simulink model "Nugraha_Setya_Ardi_10714522_952033"  (R2020b)
settings: Solver=ode15s  StartTime=0.0  StopTime=1000
undefined symbols (not defined in the file): deg, s
libraries: sharedtransform x1
settings Model: SimulationMode=rapid-accelerator  Creator=nugra  LastModifiedBy=nugra
settings SolverCC: ZeroCrossAlgorithm=Adaptive

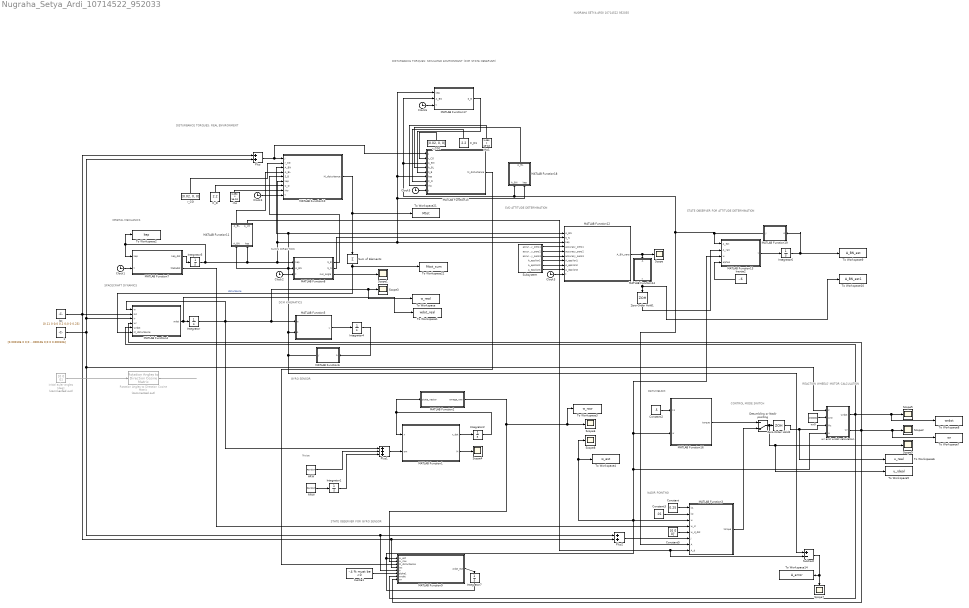
== system Nugraha_Setya_Ardi_10714522_952033 ==
  note: Noise
  note: GYRO SENSOR
  note: NADIR POINTNG
  note: DETUMBLING
  note: REACTION WHEELS'
      | MOTOR CALCULATION
  note: DCM KINEMATICS
  note: DISTURBANCE TORQUES:
      | REAL ENVIRONMENT
  note: ORBITAL MECHANICS
  note: SUN'S DIRECTION
  note: SPACECRAFT DYNAMICS
  note: CONTROL MODE
      | SWITCH
  note: STATE OBSERVER FOR
      | GYRO SENSOR
  note: STATE OBSERVER FOR
      | ATTITUDE DETERMINATION
  note: DISTURBANCE TORQUES:
      | SIMULATED ENVIRONMENT
      | (FOR STATE OBSERVER)
  note: NUGRAHA SETYA ARDI
      | 10714522
      | 952035
  note: SVD ATTITUDE DETERMINATION
  ARW : RandomNumber  Variance=(1/4*deg2rad([0.2 0.2 0.2]/sqrt(3600))).^2 %[0.2 deg/s^.5]  SampleTime=1/1000
  C_D : Constant  Value=2.2
  C_D1 : Constant  Value=2.2
  Clock{1..6} (6 alike) : Clock
  Constant : Constant  Value=0.25
  Constant2 : Constant  Value=.5
  Constant3 : Constant  Value=.01
  Constant5 : Constant  Value=[0 0 0]'
  Detumbling or Nadir pointing : ManualSwitch  CurrentSetting=0
  Inertia1 : Constant  Value=-.4 % must be <0
  Inertia2 : Constant  Value=-.6
  Integrator : Integrator  InitialCondition=deg2rad([5 10 -7])
  Integrator1 : Integrator  InitialCondition=[1/3600 1/3600 1/3600] % [deg/s], i.e. 1 deg/hour
  Integrator2 : Integrator  InitialCondition=[0 0 0 0 0 0]'
  Integrator4 : Integrator  InitialCondition=eye(3,3)
  Integrator5 : Integrator  InitialCondition=[7500, 0.1, deg2rad(10), deg2rad(40), deg2rad(60), 0]
  Integrator6 : Integrator  InitialCondition=zeros(3,3)
  Integrator7 : Integrator  InitialCondition=[0 0 0]
  Ir : Constant  Value=[0.000106 0 0;0 0.000106 0;0 0 0.000106]  VectorParams1D=off
  Isc : Constant  Value=[0.11 0 0;0 0.2 0;0 0 0.23]  VectorParams1D=off
  MATLAB Function1 : MATLAB Function  TreatAsAtomicUnit=on
  MATLAB Function10 : MATLAB Function  TreatAsAtomicUnit=on
  MATLAB Function11 : MATLAB Function  TreatAsAtomicUnit=on
  MATLAB Function12 : MATLAB Function  TreatAsAtomicUnit=on
  MATLAB Function13 : MATLAB Function  TreatAsAtomicUnit=on
  MATLAB Function14 : MATLAB Function  TreatAsAtomicUnit=on
  MATLAB Function15 : MATLAB Function  TreatAsAtomicUnit=on
  MATLAB Function16 : MATLAB Function  TreatAsAtomicUnit=on
  MATLAB Function17 : MATLAB Function  TreatAsAtomicUnit=on
  MATLAB Function18 : MATLAB Function  TreatAsAtomicUnit=on
  MATLAB Function19 : MATLAB Function  TreatAsAtomicUnit=on
  MATLAB Function2 : MATLAB Function  TreatAsAtomicUnit=on
  MATLAB Function3 : MATLAB Function  TreatAsAtomicUnit=on
  MATLAB Function4 : MATLAB Function  TreatAsAtomicUnit=on
  MATLAB Function5 : MATLAB Function  TreatAsAtomicUnit=on
  MATLAB Function6 : MATLAB Function  TreatAsAtomicUnit=on
  MATLAB Function7 : MATLAB Function  TreatAsAtomicUnit=on
  MATLAB Function8 : MATLAB Function  TreatAsAtomicUnit=on
  MATLAB Function9 : MATLAB Function  TreatAsAtomicUnit=on
  Plus : Sum
  Plus1 : Sum  Inputs=+++
  Plus2 : Sum
  RRW : RandomNumber  Variance=(1/4*deg2rad([0.3 0.3 0.3]/3600)).^2 % [0.3 deg/s^1.5]  SampleTime=1/1000
  Rotation Angles to Direction Cosine Matrix : sharedtransform/Rotation Angles to Direction Cosine Matrix  Commented=on  rotationOrder=XYZ  aMode=aMode
      settings: SourceProductBaseCode=AE,PW,MT,UV,VE,VP
  Scope{,1..9} (10 alike) : Scope
  Subsystem : Subsystem
  Subtract : Sum  Inputs=+-
  Sum of Elements : Sum  Inputs=+  CollapseMode=Specified dimension  CollapseDim=2
  To Workspace : ToWorkspace  VariableName=w_real  SaveFormat=Structure With Time  SampleTime=-1
  To Workspace1 : ToWorkspace  VariableName=wdot_real  SaveFormat=Structure With Time  SampleTime=-1
  To Workspace10 : ToWorkspace  VariableName=A_BN_est1  SaveFormat=Timeseries  SampleTime=-1
  To Workspace14 : ToWorkspace  VariableName=A_error  SaveFormat=Structure With Time  SampleTime=-1
  To Workspace2 : ToWorkspace  VariableName=kep  SaveFormat=Timeseries  SampleTime=-1
  To Workspace21 : ToWorkspace  VariableName=Mtot  SaveFormat=Structure With Time  SampleTime=-1
  To Workspace22 : ToWorkspace  VariableName=Mtot_sum  SaveFormat=Structure With Time  SampleTime=-1
  To Workspace3 : ToWorkspace  VariableName=w_raw  SaveFormat=Structure With Time  SampleTime=-1
  To Workspace4 : ToWorkspace  VariableName=w_est  SaveFormat=Structure With Time  SampleTime=-1
  To Workspace5 : ToWorkspace  VariableName=u_ideal  SaveFormat=Structure With Time  SampleTime=-1
  To Workspace6 : ToWorkspace  VariableName=u_real  SaveFormat=Structure With Time  SampleTime=-1
  To Workspace7 : ToWorkspace  VariableName=wr  SaveFormat=Structure With Time  SampleTime=-1
  To Workspace8 : ToWorkspace  VariableName=wrdot  SaveFormat=Structure With Time  SampleTime=-1
  To Workspace9 : ToWorkspace  VariableName=A_BN_est  SaveFormat=Timeseries  SampleTime=-1
  Zero-Order Hold1 : ZeroOrderHold  SampleTime=0.01
  Zero-Order Hold2 : ZeroOrderHold  SampleTime=0.01
  initial euler angles [deg] : Constant  Commented=on  Value=[0 0 0]
  r_CG : Constant  Value=[0.02, 0, 0]'
  r_CG1 : Constant  Value=[0.02, 0, 0]'
  rho : Constant  Value=1.454 * 1e-13
  rho1 : Constant  Value=1.454 * 1e-13
  wr and wrdot calculation : Subsystem
  wr0 : Constant  Value=[0;0;0]
  wires:
  MATLAB Function4/1(wdot) -> To Workspace1/1, Integrator/1
  Isc/1 -> Plus/1, MATLAB Function9/4(Isc), Plus2/2, MATLAB Function4/2(Isc)
  Ir/1 -> Plus2/1, MATLAB Function9/5(Ir), wr and wrdot calculation/1(Ir), Plus/2, MATLAB Function4/3(Ir)
  MATLAB Function5/1(y) -> Integrator4/1
  Integrator4/1 -> MATLAB Function6/1(A)
  Clock1/1 -> MATLAB Function7/2(t)
  MATLAB Function7/1(kep_dot) -> Integrator5/1
  Clock2/1 -> MATLAB Function8/3(t)
  Subsystem/2(accuracy_sens2) -> MATLAB Function12/5(accuracy_sens2)
  MATLAB Function6/1(y) -> Subtract/1, MATLAB Function11/1(A_BN), MATLAB Function10/3(A_BN), MATLAB Function12/1(A_BN), MATLAB Function8/2(A_BN), MATLAB Function5/2(A)
  Subsystem/1(accuracy_sens1) -> MATLAB Function12/4(accuracy_sens1)
  MATLAB Function8/2(S_N) -> MATLAB Function12/2(S_N)
  Integrator5/1 -> MATLAB Function11/2(kep), MATLAB Function8/1(kep), MATLAB Function10/6(kep), MATLAB Function12/3(kep), MATLAB Function18/2(kep), MATLAB Function17/1(kep), MATLAB Function15/6(kep), MATLAB Function7/1(kep), To Workspace2/1
  Clock3/1 -> MATLAB Function12/10(t)
  MATLAB Function8/1(S_B) -> MATLAB Function10/5(S_B)
  Clock4/1 -> MATLAB Function10/9(t)
  C_D/1 -> MATLAB Function10/7(C_D)
  rho/1 -> MATLAB Function10/8(rho)
  r_CG/1 -> MATLAB Function10/2(r_CG)
  Plus/1 -> MATLAB Function15/1(J), MATLAB Function10/1(J)
  MATLAB Function11/1(A_BL) -> MATLAB Function10/4(A_BL)
  Integrator1/1 -> Plus1/3
  MATLAB Function1/2(M) -> Scope4/1
  MATLAB Function1/1(x_dot) -> Integrator2/1
  RRW/1 -> Integrator1/1
  Integrator/1 -> MATLAB Function5/1(w), To Workspace/1, Scope3/1, Plus1/1, MATLAB Function4/1(w)
  ARW/1 -> Plus1/2
  Plus1/1 -> MATLAB Function1/2(om)
  Constant2/1 -> MATLAB Function16/1(k1)
  MATLAB Function16/1(torque) -> Detumbling or Nadir pointing/1
  wr0/1 -> wr and wrdot calculation/2(wr0)
  wr and wrdot calculation/1(wrdot) -> MATLAB Function9/7(wrdot), To Workspace8/1, Scope5/1, MATLAB Function4/5(wrdot)
  wr and wrdot calculation/2(wr) -> MATLAB Function9/8(wr), To Workspace7/1, Scope2/1, MATLAB Function4/4(wr)
  Integrator2/1 -> MATLAB Function1/1(x), MATLAB Function2/1(state_vector)
  MATLAB Function8/3(sun_angle) -> Scope1/1
  Constant/1 -> MATLAB Function3/1(k1)
  Constant3/1 -> MATLAB Function3/2(k2)
  MATLAB Function11/2(A_LN) -> Subtract/2, MATLAB Function3/8(A_d)
  MATLAB Function7/2(thetadot) -> MATLAB Function3/4(w_d)
  Constant5/1 -> MATLAB Function3/5(w_d_dot)
  MATLAB Function3/1(torque) -> Detumbling or Nadir pointing/2
  Plus2/1 -> MATLAB Function3/6(J)
  Detumbling or Nadir pointing/1 -> To Workspace5/1, Scope9/1, Zero-Order Hold2/1
  Subtract/1 -> Scope7/1, To Workspace14/1
  MATLAB Function2/1(omega_raw) -> MATLAB Function9/2(w_raw), To Workspace3/1, Scope6/1
  Zero-Order Hold1/1 -> MATLAB Function13/2(A_raw)
  Zero-Order Hold2/1 -> To Workspace6/1, wr and wrdot calculation/3(Mc)
  MATLAB Function9/1(wdot_est) -> Integrator7/1
  Inertia1/1 -> MATLAB Function9/6(alpha1)
  MATLAB Function10/1(M_disturbance) -> To Workspace21/1, Sum of Elements/1
  MATLAB Function13/1(y) -> Integrator6/1
  Inertia2/1 -> MATLAB Function13/4(alpha1)
  Clock5/1 -> MATLAB Function15/9(t)
  r_CG1/1 -> MATLAB Function15/2(r_CG)
  C_D1/1 -> MATLAB Function15/7(C_D)
  rho1/1 -> MATLAB Function15/8(rho)
  Clock6/1 -> MATLAB Function17/3(t)
  MATLAB Function17/1(S_B) -> MATLAB Function15/5(S_B)
  MATLAB Function18/1(A_BL) -> MATLAB Function15/4(A_BL)
  MATLAB Function15/1(M_disturbance) -> MATLAB Function9/3(M_disturbance)
  Subsystem/3(accuracy_sens3) -> MATLAB Function12/6(accuracy_sens3)
  Subsystem/4(A_epsilon1) -> MATLAB Function12/7(A_epsilon1)
  Subsystem/5(A_epsilon2) -> MATLAB Function12/8(A_epsilon2)
  Subsystem/6(A_epsilon3) -> MATLAB Function12/9(A_epsilon3)
  Integrator7/1 -> wr and wrdot calculation/4(w), MATLAB Function13/3(w), MATLAB Function16/2(w), MATLAB Function3/3(w), To Workspace4/1, Scope8/1, MATLAB Function9/1(w_est)
  MATLAB Function12/1(A_BN_sens) -> Scope/1, MATLAB Function14/1(A)
  Integrator6/1 -> To Workspace9/1, MATLAB Function19/1(A)
  MATLAB Function14/1(y) -> Zero-Order Hold1/1, To Workspace10/1
  Sum of Elements/1 -> MATLAB Function4/6(M_disturbance), To Workspace22/1  "disturbance"
  Rotation Angles to Direction Cosine Matrix/1 -> ?
  initial euler angles [deg]/1 -> Rotation Angles to Direction Cosine Matrix/1
  MATLAB Function19/1(y) -> MATLAB Function3/7(A), MATLAB Function18/1(A_BN), MATLAB Function17/2(A_BN), MATLAB Function15/3(A_BN), MATLAB Function13/1(A_est)

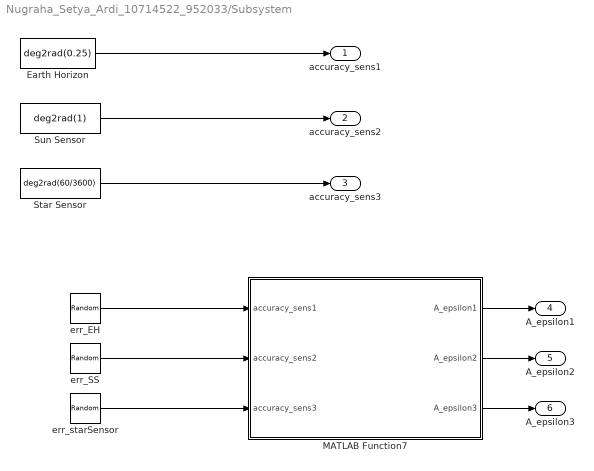
== system Nugraha_Setya_Ardi_10714522_952033/Subsystem ==
  Earth Horizon : Constant  Value=deg2rad(0.25)
  MATLAB Function7 : MATLAB Function  TreatAsAtomicUnit=on
  Star Sensor : Constant  Value=deg2rad(60/3600)
  Sun Sensor : Constant  Value=deg2rad(1)
  err_EH : RandomNumber  Variance=(1/4*deg2rad([0.25 0.25 0.25])).^2  Seed=[1 2 3]  SampleTime=1/100
  err_SS : RandomNumber  Variance=(1/4*deg2rad([1 1 1])).^2  Seed=[4 5 6]  SampleTime=1/100
  err_starSensor : RandomNumber  Variance=(1/4*deg2rad([60/3600 60/3600 60/3600])).^2  Seed=[4 5 6]  SampleTime=1/4
  accuracy_sens1 : Outport
  accuracy_sens2 : Outport  Port=2
  accuracy_sens3 : Outport  Port=3
  A_epsilon1 : Outport  Port=4
  A_epsilon2 : Outport  Port=5
  A_epsilon3 : Outport  Port=6
  wires:
  MATLAB Function7/1(A_epsilon1) -> A_epsilon1/1
  MATLAB Function7/2(A_epsilon2) -> A_epsilon2/1
  Earth Horizon/1 -> accuracy_sens1/1
  Sun Sensor/1 -> accuracy_sens2/1
  err_SS/1 -> MATLAB Function7/2(accuracy_sens2)
  err_EH/1 -> MATLAB Function7/1(accuracy_sens1)
  Star Sensor/1 -> accuracy_sens3/1
  err_starSensor/1 -> MATLAB Function7/3(accuracy_sens3)
  MATLAB Function7/3(A_epsilon3) -> A_epsilon3/1

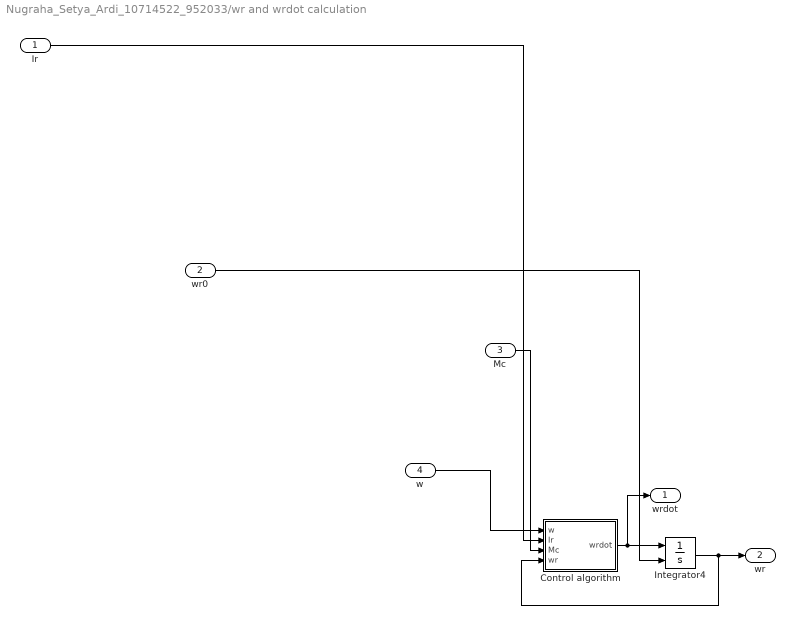
== system Nugraha_Setya_Ardi_10714522_952033/wr and wrdot calculation ==
  Ir : Inport
  wr0 : Inport  Port=2
  Mc : Inport  Port=3
  w : Inport  Port=4
  Control algorithm : MATLAB Function  TreatAsAtomicUnit=on
  Integrator4 : Integrator  InitialConditionSource=external
  wrdot : Outport
  wr : Outport  Port=2
  wires:
  Control algorithm/1(wrdot) -> wrdot/1, Integrator4/1
  Ir/1 -> Control algorithm/2(Ir)
  wr0/1 -> Integrator4/2
  Mc/1 -> Control algorithm/3(Mc)
  w/1 -> Control algorithm/1(w)
  Integrator4/1 -> Control algorithm/4(wr), wr/1

== matlab function Nugraha_Setya_Ardi_10714522_952033/MATLAB Function8 ==
  data: S_B output; S_N output; kep input; sun_angle output; A_BN input; t input
function [ S_B, S_N, sun_angle] = sun_direction(kep, A_BN, t)
% kep = [a e i om, Om, th]
a  = kep(1);
e  = kep(2);
i  = kep(3);
om = kep(4);
Om = kep(5);
th = kep(6);

R = a*(1-e^2) / (1+e*cos(th));
r_N = R * [cos(th);
           sin(th)*cos(i);
           sin(th)*sin(i)];
r_B = A_BN * r_N;

R_s = 149597870.691; % 1AU [km]
mu_s = 132712440017.987;
n_s  = sqrt(mu_s/R_s^3);

epsilon = deg2rad(23.45);
% Sun direction w.r.t. S/C ~ Sun direction w.r.t. Earth
S_N = R_s * [cos(n_s*t), sin(n_s*t)*cos(epsilon), sin(n_s*t)*sin(epsilon)]';
S_B = A_BN*S_N;

sun_angle = acos(complex(dot(r_B, S_B)/(norm(r_B)*norm(S_B))));

== matlab function Nugraha_Setya_Ardi_10714522_952033/MATLAB Function9 ==
  data: w_est input; w_raw input; M_disturbance input; wdot_est output; Isc input; Ir input; alpha1 input; wrdot input; wr input
function wdot_est = stateObserbver(w_est,w_raw,M_disturbance,Isc,Ir,alpha1,wrdot,wr)
% 
% 
% % Moments of Inertia [kg*m^2]
% % (12U Cubesat)
% J1 = J(1,1);
% J2 = J(2,2);
% J3 = J(3,3);
% 
% C1 = (J2-J3)/J1;
% C2 = (J3-J1)/J2;
% C3 = (J1-J2)/J3;
% 
% 
% w_est_dot = zeros(3,1);
% w_est_dot(1) = C1 * w_est(2)*w_est(3) + u_tot(1)/J1 + alpha1*(w_est(1) - w_raw(1));
% w_est_dot(2) = C2 * w_est(1)*w_est(3) + u_tot(2)/J2 + alpha1*(w_est(2) - w_raw(2));
% w_est_dot(3) = C3 * w_est(1)*w_est(2) + u_tot(3)/J3 + alpha1*(w_est(3) - w_raw(3));

wdot_est = inv(Isc)*(M_disturbance - cross(w_est,(Isc*w_est)) - Ir*wrdot - cross(w_est,(Ir*wr))) + alpha1*(w_est-w_raw);

== matlab function Nugraha_Setya_Ardi_10714522_952033/MATLAB Function10 ==
  data: J input; r_CG input; A_BN input; M_disturbance output; A_BL input; S_B input; kep input; C_D input; rho input; t input
function M_disturbance    = disturbanceTorques(J, r_CG, A_BN, A_BL, S_B, kep, C_D, rho, t)

G = 6.67408e-11;
m_E = 5.972e+24;
a  = kep(1);    e  = kep(2);    i = kep(3);
OM = kep(4);    om = kep(5);    th = kep(6);
R_equat = 6371e+3; % [m]
p = a*(1-e^2);
R = p / (1+e*cos(th)) * 1e+3; % [m]

% Moments of Inertia [kg*m^2]
% (12U Cubesat)
J1 = J(1,1);
J2 = J(2,2);
J3 = J(3,3);

C1 = (J2-J3)/J1;
C2 = (J3-J1)/J2;
C3 = (J1-J2)/J3;
%% Gravity Gradient Torque
c = A_BL * [1;0;0];

M_GG = [- 3*G*m_E/R^3 *C1* c(3)*c(2);
        - 3*G*m_E/R^3 *C2* c(1)*c(3);
        - 3*G*m_E/R^3 *C3* c(2)*c(1)];
                      
%% SRP Torque @ 600 Km (Direct Solar Rad. + Sun Rad. Reflected by Earth + Earth Rad.)
F_e = 1358 + 580 + 143.4; % [W/m^2]
P = F_e / (3*1e+8);

N_body = 6; % # main body surfaces
N_SP = 4; % # solar panel surfaces

U = 0.1; % 1U length

N = zeros(N_body+N_SP,3);
A = zeros(N_body+N_SP,1);
r = zeros(N_body+N_SP,3);
n1 = [1 0 0];  n2 = [0 1 0];  n3 = [0 0 1];
% S/C Main Body: Normals, Surface Coefficients, Areas
N(1,:) = n1;    N(2,:) = n2;     N(3,:) = n3;
N(4,:) = -n1;   N(5,:) = -n2;   N(6,:) = -n3;
rho_s_body = .5;     rho_d_body = .1;
A(1:N_body) = [4 8 8 4 8 8]*U^2; % [m^2]

% Solar Panels: Normals, Surface Coefficients, Areas
N(7,:) = n1;    N(8,:) = -n1;   N(9,:) = n1;    N(10,:) = -n1;
rho_s_SP = .5;     rho_d_SP = .1;
A(N_body+1:N_body+N_SP) = [8 8 8 8]*U^2; % [m^2]

% L.u.c. a RF centered @ Geometric Center of S/C::
% we will use it to define the coordinates of each surface's center
% along w/ the coordinates of th CG w.r.t. GC
r(1,:) = [2 0 0]*U;  r(2,:) = [0 1 0]*U;  r(3,:) = [0 0 1]*U;
r(4,:) = [-2 0 0]*U; r(5,:) = [0 -1 0]*U; r(6,:) = [0 0 -1]*U;
r(7,:) = [-2 3 0]*U;   r(8,:)  = [-2 -3 0]*U;
r(9,:) = [-2 3 0]*U;   r(10,:) = [-2 -3 0]*U;

S_B_norm = S_B / norm(S_B);

M_SRP = zeros(3,1);
for k = 1:N_body+N_SP
    if k <= N_body
        rho_s = rho_s_body;     rho_d = rho_d_body;
    else
        rho_s = rho_s_SP;       rho_d = rho_d_SP;
    end
    
    n_k = N(k,:)';
    F_k = - P*A(k)*dot(S_B_norm,n_k) * ( (1-rho_s)*S_B_norm + (2*rho_s*dot(S_B_norm,n_k)+2/3*rho_d)*n_k );
    
    if dot(S_B_norm, n_k) > 0
        r_k = (r(k,:) - r_CG')';
        M_SRP_k = cross(r_k, F_k);
    else
        M_SRP_k = zeros(3,1);
    end
    
    M_SRP = M_SRP + M_SRP_k;
        
end

%% Air-Drag Torque

w_E = 2*pi/(23*3600 + 56*60 + 4.09); % Earth's angular rate [rad/s]
mu_E = 398600.433; % [km^3/s^2]



% Rotation matrices: Earth-Centered Inertial --> Perifocal   (ECI->PF)
R_om = [cos(om)  sin(om)    0   ;
        -sin(om) cos(om)    0   ;
           0        0       1   ];
       
R_i  = [   1        0       0   ;
           0     cos(i)   sin(i);
           0    -sin(i)   cos(i)];
       
R_OM = [cos(OM)  sin(OM)    0   ;
        -sin(OM) cos(OM)    0   ;
           0        0       1   ];
    
R313 = R_om * R_i * R_OM; % ECI --> PF


R_PF = R * [cos(th), sin(th), 0]';
v_PF = sqrt(mu_E/p) * [-sin(th), (e+cos(th)), 0]';
% PF --> ECI
r_ECI = R313'* R_PF;
v_ECI = R313'* v_PF;


v_rel_N = v_ECI + cross([0 0 w_E]', r_ECI);

v_rel_B = A_BN*v_rel_N; % Relative atmosphere velocity (@body frame)
v_rel_B_unit = v_rel_B / norm(v_rel_B);


M_drag = zeros(3,1);
for k = 1:N_body+N_SP
    
    n_k = N(k,:)';
    F_k = - .5 * C_D * rho * norm(v_rel_B)^2 * dot(n_k,v_rel_B_unit) * A(k) * v_rel_B_unit;
    
    
    if dot(S_B_norm, n_k) > 0
        r_k = (r(k,:) - r_CG')';
        M_drag_k = cross(r_k, F_k);
    else
        M_drag_k = zeros(3,1);
    end
    
    M_drag = M_drag + M_drag_k;
        
end

%% Magnetic Torque
g10 = -29615e-9;  g11 = -1728e-9;   h11 = 5186e-9;
H0 = sqrt(g10^2 + g11^2 + h11^2);
m = [sind(11.5)*cos(w_E*t);
     sind(11.5)*sin(w_E*t);
     cosd(11.5)];
r_N = R * [cos(th);
           sin(th)*cos(i);
           sin(th)*sin(i)];
       
% Magnetic field vector
b_N = R_equat^3*H0/R^3 * (3*dot(m/norm(m),r_N/norm(r_N))*r_N/norm(r_N) - m/norm(m));
b_B = A_BN * b_N;

% Parasitic magnetic torque
M_magn = cross(m, b_B);

M_disturbance = [M_SRP(:), M_magn(:), M_GG(:)];

== matlab function Nugraha_Setya_Ardi_10714522_952033/MATLAB Function11 ==
  data: A_BN input; A_BL output; kep input; A_LN output
function [A_BL, A_LN] = fcn(A_BN, kep)

i  = kep(3);
Om = kep(4)
w = kep(5);
th = kep(6);


A_1 = [ cos(th+w) sin(th+w) 0;
        -sin(th+w) cos(th+w) 0;
          0         0    1];
A_2 = [1      0     0;
       0   cos(i) sin(i);
       0  -sin(i) cos(i)];
A_3 = [cos(Om) sin(Om) 0;-sin(Om) cos(Om) 0;0 0 1];
A_LN = A_1*A_2*A_3;

A_BL = A_BN*A_LN';

== matlab function Nugraha_Setya_Ardi_10714522_952033/MATLAB Function12 ==
  data: A_BN input; A_BN_sens output; S_N input; kep input; accuracy_sens1 input; accuracy_sens2 input; accuracy_sens3 input; A_epsilon1 input; A_epsilon2 input; A_epsilon3 input; t input
function A_BN_sens = sensorModel(A_BN, S_N, kep, accuracy_sens1, accuracy_sens2,accuracy_sens3, A_epsilon1, A_epsilon2,A_epsilon3, t)

i = kep(3);
th = kep(6);

r_N =      [cos(th);
           sin(th)*cos(i);
           sin(th)*sin(i)]; % unit vector that identifies S/C's position w.r.t.
                            % inertial frame centered at Earth
                            
S_N = S_N / norm(S_N);  % unit vector that identifies Sun direction in the
                        % inertial frame
v_N1 = r_N;     
v_N2 = S_N;
v_N3 = [1;0;0]          % fixed star for star sensor
v_B1 = A_epsilon1 * A_BN * v_N1;
v_B2 = A_epsilon2 * A_BN * v_N2;
v_B3 = A_epsilon3 * A_BN * v_N3;

%% SVD algorithm for attitude estimation
prec_sens1 = 1/norm(accuracy_sens1);
prec_sens2 = 1/norm(accuracy_sens2);
prec_sens3 = 1/norm(accuracy_sens3);
alpha = [prec_sens1 prec_sens2 prec_sens3] / (prec_sens1+prec_sens2+prec_sens3); % s.t. sum(alpha) = 1
B = alpha(1)*v_B1*v_N1' + alpha(2)*v_B2*v_N2' + alpha(3)*v_B3*v_N3';
[U,~,V] = svd(B);
M = diag([1, 1, det(U)*det(V)]);
A_BN_sens = U*M*V';

== matlab function Nugraha_Setya_Ardi_10714522_952033/Subsystem/MATLAB Function7 ==
  data: accuracy_sens1 input; A_epsilon1 output; accuracy_sens2 input; A_epsilon2 output; accuracy_sens3 input; A_epsilon3 output
function [A_epsilon1, A_epsilon2, A_epsilon3] = sensor_error(accuracy_sens1, accuracy_sens2, accuracy_sens3)


psi_acc = accuracy_sens1(1);
th_acc  = accuracy_sens1(2);
phi_acc = accuracy_sens1(3);
A_epsilon1 = [cos(psi_acc)*cos(th_acc)  (cos(psi_acc)*sin(th_acc)*sin(phi_acc)+sin(psi_acc)*cos(phi_acc)) (-cos(psi_acc)*sin(th_acc)*cos(phi_acc)+sin(psi_acc)*sin(phi_acc));
                -sin(psi_acc)*cos(th_acc) (-sin(psi_acc)*sin(th_acc)*sin(phi_acc)+cos(psi_acc)*cos(phi_acc))  (sin(psi_acc)*sin(th_acc)*cos(phi_acc)+cos(psi_acc)*sin(phi_acc));
                 sin(th_acc)               -cos(th_acc)*sin(phi_acc)                                           cos(th_acc)*cos(phi_acc)];
             
             

psi_acc = accuracy_sens2(1);
th_acc  = accuracy_sens2(2);
phi_acc = accuracy_sens2(3);
A_epsilon2 = [cos(psi_acc)*cos(th_acc)  (cos(psi_acc)*sin(th_acc)*sin(phi_acc)+sin(psi_acc)*cos(phi_acc)) (-cos(psi_acc)*sin(th_acc)*cos(phi_acc)+sin(psi_acc)*sin(phi_acc));
                -sin(psi_acc)*cos(th_acc) (-sin(psi_acc)*sin(th_acc)*sin(phi_acc)+cos(psi_acc)*cos(phi_acc))  (sin(psi_acc)*sin(th_acc)*cos(phi_acc)+cos(psi_acc)*sin(phi_acc));
                 sin(th_acc)               -cos(th_acc)*sin(phi_acc)                                           cos(th_acc)*cos(phi_acc)];


             
psi_acc = accuracy_sens3(1);
th_acc  = accuracy_sens3(2);
phi_acc = accuracy_sens3(3);
A_epsilon3 = [cos(psi_acc)*cos(th_acc)  (cos(psi_acc)*sin(th_acc)*sin(phi_acc)+sin(psi_acc)*cos(phi_acc)) (-cos(psi_acc)*sin(th_acc)*cos(phi_acc)+sin(psi_acc)*sin(phi_acc));
                -sin(psi_acc)*cos(th_acc) (-sin(psi_acc)*sin(th_acc)*sin(phi_acc)+cos(psi_acc)*cos(phi_acc))  (sin(psi_acc)*sin(th_acc)*cos(phi_acc)+cos(psi_acc)*sin(phi_acc));
                 sin(th_acc)               -cos(th_acc)*sin(phi_acc)                                           cos(th_acc)*cos(phi_acc)];
end

== matlab function Nugraha_Setya_Ardi_10714522_952033/MATLAB Function13 ==
  data: A_est input; A_raw input; w input; y output; alpha1 input
function y = stateObserbver(A_est, A_raw, w, alpha1)
W = [0,    -w(3),  w(2);
     w(3),   0,   -w(1);
    -w(2),  w(1),   0];

A_est_dot = -W * A_est + alpha1*(A_est-A_raw);

y = A_est_dot;

== matlab function Nugraha_Setya_Ardi_10714522_952033/MATLAB Function14 ==
  data: A input; y output
function y = orthonorm(A)

% Recall: for a matrix to be orthonormal it is necessary that
%         det(A)=1  -->  tr(A'A - I) = 0

tol = 1e-7;
k = 0;
while trace(A'*A - eye(3,3)) > tol
    k = k+1;
    A = 3/2 * A - 1/2 * A*A'*A;
end

y = A;

== matlab function Nugraha_Setya_Ardi_10714522_952033/MATLAB Function15 ==
  data: J input; r_CG input; A_BN input; M_disturbance output; A_BL input; S_B input; kep input; C_D input; rho input; t input
function M_disturbance  = disturbanceTorques(J, r_CG, A_BN, A_BL, S_B, kep, C_D, rho, t)

G = 6.67408e-11;
m_E = 5.972e+24;
a  = kep(1);    e  = kep(2);    i = kep(3);
OM = kep(4);    om = kep(5);    th = kep(6);
R_equat = 6371e+3; % [m]
p = a*(1-e^2);
R = p / (1+e*cos(th)) * 1e+3; % [m]

% Moments of Inertia [kg*m^2]
% (12U Cubesat)
J1 = J(1,1);
J2 = J(2,2);
J3 = J(3,3);

C1 = (J2-J3)/J1;
C2 = (J3-J1)/J2;
C3 = (J1-J2)/J3;
%% Gravity Gradient Torque
c = A_BL * [1;0;0];

M_GG = [- 3*G*m_E/R^3 *C1* c(3)*c(2);
        - 3*G*m_E/R^3 *C2* c(1)*c(3);
        - 3*G*m_E/R^3 *C3* c(2)*c(1)];
                      
%% SRP Torque @ 600 Km (Direct Solar Rad. + Sun Rad. Reflected by Earth + Earth Rad.)
F_e = 1358 + 580 + 143.4; % [W/m^2]
P = F_e / (3*1e+8);

N_body = 6; % # main body surfaces
N_SP = 4; % # solar panel surfaces

U = 0.1; % 1U length

N = zeros(N_body+N_SP,3);
A = zeros(N_body+N_SP,1);
r = zeros(N_body+N_SP,3);
n1 = [1 0 0];  n2 = [0 1 0];  n3 = [0 0 1];
% S/C Main Body: Normals, Surface Coefficients, Areas
N(1,:) = n1;    N(2,:) = n2;     N(3,:) = n3;
N(4,:) = -n1;   N(5,:) = -n2;   N(6,:) = -n3;
rho_s_body = .5;     rho_d_body = .1;
A(1:N_body) = [2 3 6 2 3 6]*U^2; % [m^2]

% Solar Panels: Normals, Surface Coefficients, Areas
N(7,:) = n1;    N(8,:) = -n1;   N(9,:) = n1;    N(10,:) = -n1;
rho_s_SP = .5;     rho_d_SP = .1;
A(N_body+1:N_body+N_SP) = [6 6 6 6]*U^2; % [m^2]

% L.u.c. a RF centered @ Geometric Center of S/C::
% we will use it to define the coordinates of each surface's center
% along w/ the coordinates of th CG w.r.t. GC
r(1,:) = [1.5 0 0]*U;  r(2,:) = [0 1 0]*U;  r(3,:) = [0 0 .5]*U;
r(4,:) = [-1.5 0 0]*U; r(5,:) = [0 -1 0]*U; r(6,:) = [0 0 -.5]*U;
r(7,:) = [-1.5 2.5 0]*U;   r(8,:)  = [-1.5 -2.5 0]*U;
r(9,:) = [-1.5 2.5 0]*U;   r(10,:) = [-1.5 -2.5 0]*U;

S_B_norm = S_B / norm(S_B);

M_SRP = zeros(3,1);
for k = 1:N_body+N_SP
    if k <= N_body
        rho_s = rho_s_body;     rho_d = rho_d_body;
    else
        rho_s = rho_s_SP;       rho_d = rho_d_SP;
    end
    
    n_k = N(k,:)';
    F_k = - P*A(k)*dot(S_B_norm,n_k) * ( (1-rho_s)*S_B_norm + (2*rho_s*dot(S_B_norm,n_k)+2/3*rho_d)*n_k );
    
    if dot(S_B_norm, n_k) > 0
        r_k = (r(k,:) - r_CG')';
        M_SRP_k = cross(r_k, F_k);
    else
        M_SRP_k = zeros(3,1);
    end
    
    M_SRP = M_SRP + M_SRP_k;
        
end

%% Air-Drag Torque

w_E = 2*pi/(23*3600 + 56*60 + 4.09); % Earth's angular rate [rad/s]
mu_E = 398600.433; % [km^3/s^2]



% Rotation matrices: Earth-Centered Inertial --> Perifocal   (ECI->PF)
R_om = [cos(om)  sin(om)    0   ;
        -sin(om) cos(om)    0   ;
           0        0       1   ];
       
R_i  = [   1        0       0   ;
           0     cos(i)   sin(i);
           0    -sin(i)   cos(i)];
       
R_OM = [cos(OM)  sin(OM)    0   ;
        -sin(OM) cos(OM)    0   ;
           0        0       1   ];
    
R313 = R_om * R_i * R_OM; % ECI --> PF


R_PF = R * [cos(th), sin(th), 0]';
v_PF = sqrt(mu_E/p) * [-sin(th), (e+cos(th)), 0]';
% PF --> ECI
r_ECI = R313'* R_PF;
v_ECI = R313'* v_PF;


v_rel_N = v_ECI + cross([0 0 w_E]', r_ECI);

v_rel_B = A_BN*v_rel_N; % Relative atmosphere velocity (@body frame)
v_rel_B_unit = v_rel_B / norm(v_rel_B);


M_drag = zeros(3,1);
for k = 1:N_body+N_SP
    
    n_k = N(k,:)';
    F_k = - .5 * C_D * rho * norm(v_rel_B)^2 * dot(n_k,v_rel_B_unit) * A(k) * v_rel_B_unit;
    
    
    if dot(S_B_norm, n_k) > 0
        r_k = (r(k,:) - r_CG')';
        M_drag_k = cross(r_k, F_k);
    else
        M_drag_k = zeros(3,1);
    end
    
    M_drag = M_drag + M_drag_k;
        
end

%% Magnetic Torque
g10 = -29615e-9;  g11 = -1728e-9;   h11 = 5186e-9;
H0 = sqrt(g10^2 + g11^2 + h11^2);
m = [sind(11.5)*cos(w_E*t);
     sind(11.5)*sin(w_E*t);
     cosd(11.5)];
r_N = R * [cos(th);
           sin(th)*cos(i);
           sin(th)*sin(i)];
       
% Magnetic field vector
b_N = R_equat^3*H0/R^3 * (3*dot(m/norm(m),r_N/norm(r_N))*r_N/norm(r_N) - m/norm(m));
b_B = A_BN * b_N;

% Parasitic magnetic torque
M_magn = cross(m, b_B);

%%
M_disturbance = [M_drag + M_SRP + M_magn + M_GG];

== matlab function Nugraha_Setya_Ardi_10714522_952033/MATLAB Function17 ==
  data: S_B output; kep input; A_BN input; t input
function S_B  = sun_direction(kep, A_BN, t)
% kep = [a e i om, Om, th]
a  = kep(1);
e  = kep(2);
i  = kep(3);
om = kep(4);
Om = kep(5);
th = kep(6);

R = a*(1-e^2) / (1+e*cos(th));
r_N = R * [cos(th);
           sin(th)*cos(i);
           sin(th)*sin(i)];
r_B = A_BN * r_N;

R_s = 149597870.691; % 1AU [km]
mu_s = 132712440017.987;
n_s  = sqrt(mu_s/R_s^3);

epsilon = deg2rad(23.45);
% Sun direction w.r.t. S/C ~ Sun direction w.r.t. Earth
S_N = R_s * [cos(n_s*t), sin(n_s*t)*cos(epsilon), sin(n_s*t)*sin(epsilon)]';
S_B = A_BN*S_N;

sun_angle = acos(complex(dot(r_B, S_B)/(norm(r_B)*norm(S_B))));

== matlab function Nugraha_Setya_Ardi_10714522_952033/MATLAB Function18 ==
  data: A_BN input; A_BL output; kep input
function A_BL  = fcn(A_BN, kep)

i  = kep(3);
Om = kep(4)
w = kep(5);
th = kep(6);


A_1 = [ cos(th+w) sin(th+w) 0;
        -sin(th+w) cos(th+w) 0;
          0         0    1];
A_2 = [1      0     0;
       0   cos(i) sin(i);
       0  -sin(i) cos(i)];
A_3 = [cos(Om) sin(Om) 0;-sin(Om) cos(Om) 0;0 0 1];
A_LN = A_1*A_2*A_3;

A_BL = A_BN*A_LN';

== matlab function Nugraha_Setya_Ardi_10714522_952033/MATLAB Function19 ==
  data: A input; y output
function y = orthonorm(A)

% Orthonormalization: for a matrix to be orthonormal it is necessary that
%det(A)=1  -->  tr(A'A - I) = 0
tol = 1e-7;
k = 0;
while trace(A'*A - eye(3,3)) > tol
    k = k+1;
    A = 3/2 * A - 1/2 * A*A'*A;
end

y = A;

== matlab function Nugraha_Setya_Ardi_10714522_952033/MATLAB Function16 ==
  data: k1 input; torque output; w input
function torque = ideal_deTumbling(k1, w)



torque = -k1*w;


end

== matlab function Nugraha_Setya_Ardi_10714522_952033/wr and wrdot calculation/Control algorithm ==
  data: w input; Ir input; Mc input; wrdot output; wr input
function wrdot = fcn(w,Ir,Mc,wr)
wrdot = inv(Ir)*(-Mc-cross(w,(Ir*wr)));

== matlab function Nugraha_Setya_Ardi_10714522_952033/MATLAB Function1 ==
  data: x input; om input; x_dot output; M output
function [x_dot,M]  = GyroModel(x,om)
%gyro inertia parameters 
Ir = 1e-7; 
Jz = 2e-7;
%tuning parameter for visco-elastic reaction torque
k=10;
%tuning law for c for fastest convergence
c_gyro = 2*sqrt(k*Jz); 
om_x = om(1); 
om_y = om(2); 
om_z = om(3); 
%angular velocity of gyro wheel (100 deg/s)
om_r = 100*pi/180;

% defining the theta_i and \dot theta_i 
x_dot = zeros(6,1); 

th_x = x(1); 
th_y = x(2); 
th_z = x(3);
va_x = x(4);
va_y = x(5); 
va_z = x(6); 
%3 gyro dynamics expressed as 1st order differential equation
x_dot(1) = va_x;
x_dot(2) = va_y; 
x_dot(3) = va_z;
x_dot(4) = -(c_gyro/Jz)*va_x-(k/Jz)*th_x-(Ir/Jz)*om_r*om_x;
x_dot(5) = -(c_gyro/Jz)*va_y-(k/Jz)*th_y-(Ir/Jz)*om_r*om_y;
x_dot(6) = -(c_gyro/Jz)*va_z-(k/Jz)*th_z-(Ir/Jz)*om_r*om_z;
%gyro outputs 
x_dot=[x_dot(1) x_dot(2) x_dot(3) x_dot(4) x_dot(5) x_dot(6)]';

%feedback torque applied to the gyros 
M_x = -k*th_x-c_gyro*va_x;
M_y = -k*th_y-c_gyro*va_y;
M_z = -k*th_z-c_gyro*va_z;

M = [M_x M_y M_z]'; 


end

== matlab function Nugraha_Setya_Ardi_10714522_952033/MATLAB Function4 ==
  data: w input; Isc input; Ir input; wdot output; wr input; wrdot input; M_disturbance input
function wdot  = euler_eqs(w,Isc,Ir, wr,wrdot,M_disturbance)
wdot = inv(Isc)*(M_disturbance - cross(w,(Isc*w)) - Ir*wrdot - cross(w,(Ir*wr)));

== matlab function Nugraha_Setya_Ardi_10714522_952033/MATLAB Function5 ==
  data: w input; A input; y output
function y = DCM(w, A)
W = [0,    -w(3),  w(2);
     w(3),   0,   -w(1);
    -w(2),  w(1),   0];
A_dot = -W * A;
y = A_dot;

== matlab function Nugraha_Setya_Ardi_10714522_952033/MATLAB Function3 ==
  data: k1 input; k2 input; torque output; w input; w_d input; w_d_dot input; J input; A input; A_d input
function torque = ideal_tracking(k1, k2, w, w_d, w_d_dot, J, A, A_d)

A_e = A*A_d';
w_e = w - A_e*w_d;
screwSymm = A_e' - A_e;
screwSymm_invHat = [-screwSymm(2,3) screwSymm(1,3) -screwSymm(1,2)]';
torque = -k1*w_e - k2*screwSymm_invHat + cross(w,J*w) + J*(A_e*w_d_dot-cross(w_e,A_e*w_d));
end

== matlab function Nugraha_Setya_Ardi_10714522_952033/MATLAB Function2 ==
  data: state_vector input; omega_raw output
function omega_raw = fcn(state_vector)

theta_vec = state_vector(1:3);
Ir = 1e-7; 
k = 10;
om_r = 100*pi/180;

omega_raw = - k*theta_vec / (Ir*om_r);

end

== matlab function Nugraha_Setya_Ardi_10714522_952033/MATLAB Function6 ==
  data: A input; y output
function y = orthonorm(A)

% Orthonormalization: for a matrix to be orthonormal it is necessary that
%det(A)=1  -->  tr(A'A - I) = 0
tol = 1e-7;
k = 0;
while trace(A'*A - eye(3,3)) > tol
    k = k+1;
    A = 3/2 * A - 1/2 * A*A'*A;
end

y = A;

== matlab function Nugraha_Setya_Ardi_10714522_952033/MATLAB Function7 ==
  data: kep input; t input; kep_dot output; thetadot output
function [kep_dot,thetadot] = orbit_propagator(kep, t)

% kep = [a e i om, Om, th]
a  = kep(1);
e  = kep(2);
th = kep(6);

mu_e = 398600.433; % [km^3/s^2]
n = sqrt(mu_e/a^3);

kep_dot = zeros(6,1);
kep_dot(6) = n*(1+e*cos(th))^2 / ((1-e^2)^1.5);
thetadot = [0;0;kep_dot(6)];
